simulink model "followtrajectory"  (R2022b)
settings: Solver=VariableStepAuto  StartTime=0.0  StopTime=10.0  RelTol=1e-3
libraries: robotmobilelib x1
settings Model: Creator=hp  LastModifiedBy=hp

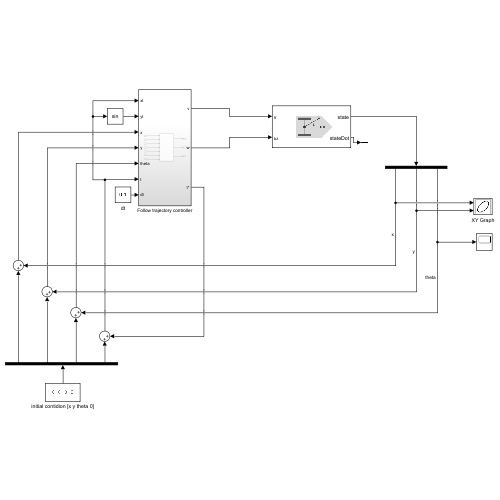
[thumbnail: Simulink's stored preview of the top-level diagram]
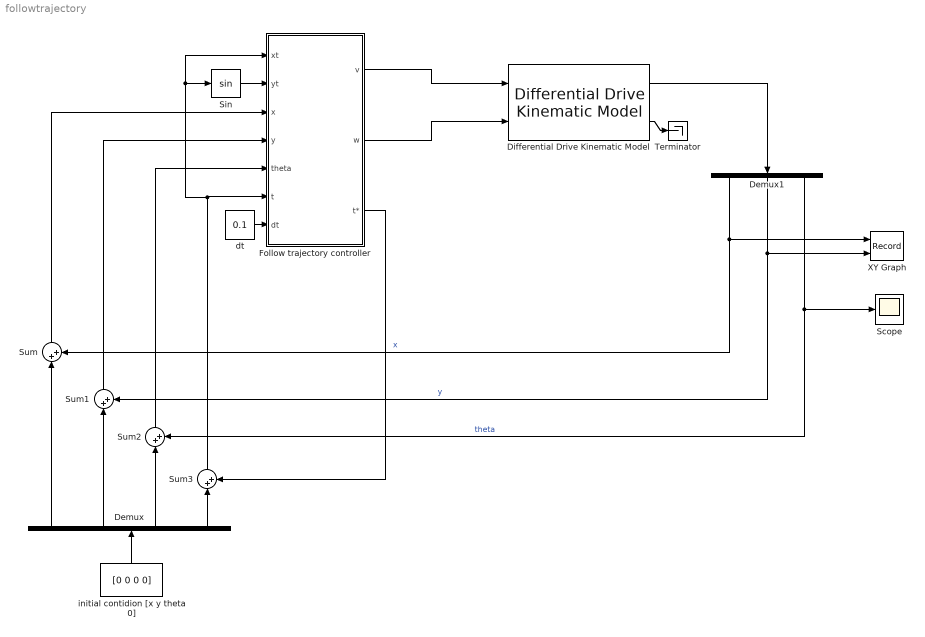
== system followtrajectory ==
  Demux : Demux
  Demux1 : Demux  Outputs=3
  Differential Drive Kinematic Model : robotmobilelib/Differential Drive Kinematic Model  VehicleInputs=Vehicle Speed & Heading Angular Velocity  WheelRadius=0.05  WheelSpeedRange=[-inf inf]  TrackWidth=0.35  InitialState=[0; 0; 0]  SimulateUsing=Interpreted execution
  Follow trajectory controller : Subsystem
  Scope : Scope
  Sin : Trigonometry
  Sum{,1..3} (4 alike) : Sum  Inputs=|++
  Terminator : Terminator
  XY Graph : Record  FileSettingsInternal="{\"entries\":[{\"content\":{\"excelSettings\":{\"content\":{},\"type\":\"Streamout.ExcelSettings\"}},\"type\":\"Streamout.FileSettingStorage\",\"uuid\":\"fe540847-13db-430f-a3f9-43ab5f5fba02\"}],\"packageUris\":[\"http://schema.mathworks.com/mf0/streamout_blocks/R2020a\"],\"version\":\"1.0\"}"  Layout=[1 1]  SignalsInternal="{\"entries\":[{\"content\":{\"signals\":[{\"content\":{\"blockPath\":[\"followtrajectory/XY Graph\"],\"channel\":[],\"dimensions\":[1],\"domain\":\"followtrajectory/XY Graph\",\"lineColor\":\"#a2142f\",\"plots\":[1],\"port\":1,\"sid\":[\"\"],\"signalID\":61,\"signalName\":\"x\"},\"type\":\"RecordBlkView.Signal\",\"uuid\":\"e5278b7b-a4bb-4301-85b3-8e4fea13731b\"},{\"content\":{\"blockPath\":[\"followtrajectory/XY Graph\"],\"channel\":[],\"dimensions\":[1],\"domain\":\"followtrajectory/XY Graph\",\"lineColor\":\"#139fff\",\"plots\":[1],\"port\":2,\"sid\":[\"\"],\"signalID\":65,\"signalName\":\"y\"},\"type\":\"RecordBlkView.Signal\",\"uuid\":\"e49be718-dbc1-456e-9503-dbe46247d26a\"}]},\"type\":\"RecordBlkView.InputSignals\",\"uuid\":\"734c241f-ef99-469e-9d0b-6cb9b84b9d56\"}],\"packageUris\":[\"http://schema.mathworks.com/mf0/streamout_blocks/R2020a\"],\"version\":\"1.0\"}"  VisualizationBindings="{\"xyplotplugin\":{\"info\":[{\"series\":[{\"bindingParametersList\":[{\"parameter\":\"X-Axis\",\"signalID\":61,\"signalName\":\"x\"},{\"parameter\":\"Y-Axis\",\"signalID\":65,\"signalName\":\"y\"}],\"seriesID\":15823}],\"subplotID\":1}]}}"  CompatibilityTag=XY
  dt : Constant  Value=0.1
  initial contidion [x y theta 0] : Constant  Value=[0 0 0 0]
  wires:
  Differential Drive Kinematic Model/2 -> Terminator/1
  Follow trajectory controller/1(v) -> Differential Drive Kinematic Model/1
  Follow trajectory controller/2(w) -> Differential Drive Kinematic Model/2
  initial contidion [x y theta 0]/1 -> Demux/1
  Differential Drive Kinematic Model/1 -> Demux1/1
  Demux/1 -> Sum/1
  Demux/2 -> Sum1/1
  Demux/3 -> Sum2/1
  Demux1/1 -> XY Graph/1, Sum/2  "x"
  Demux1/2 -> XY Graph/2, Sum1/2  "y"
  Demux1/3 -> Scope/1, Sum2/2  "theta"
  Sum/1 -> Follow trajectory controller/3(x)
  Sum1/1 -> Follow trajectory controller/4(y)
  Sum2/1 -> Follow trajectory controller/5(theta)
  dt/1 -> Follow trajectory controller/7(dt)
  Sin/1 -> Follow trajectory controller/2(yt)
  Demux/4 -> Sum3/1
  Follow trajectory controller/3(t*) -> Sum3/2
  Sum3/1 -> Follow trajectory controller/1(xt), Sin/1, Follow trajectory controller/6(t)

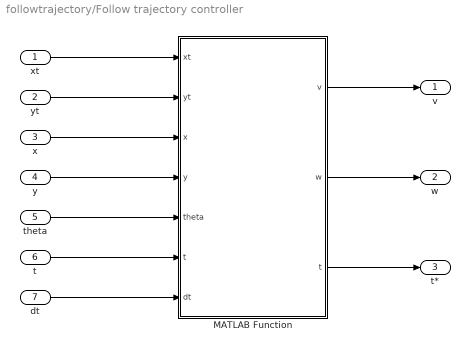
== system followtrajectory/Follow trajectory controller ==
  xt : Inport
  yt : Inport  Port=2
  x : Inport  Port=3
  y : Inport  Port=4
  theta : Inport  Port=5
  t : Inport  Port=6
  dt : Inport  Port=7
  MATLAB Function : MATLAB Function  TreatAsAtomicUnit=on
  v : Outport
  w : Outport  Port=2
  t* : Outport  Port=3
  wires:
  xt/1 -> MATLAB Function/1(xt)
  yt/1 -> MATLAB Function/2(yt)
  x/1 -> MATLAB Function/3(x)
  y/1 -> MATLAB Function/4(y)
  theta/1 -> MATLAB Function/5(theta)
  t/1 -> MATLAB Function/6("t ")
  dt/1 -> MATLAB Function/7(dt)
  MATLAB Function/1(v) -> v/1
  MATLAB Function/2(w) -> w/1
  MATLAB Function/3(t) -> t*/1

== matlab function followtrajectory/Follow trajectory controller/MATLAB Function ==
  data: xt input; v output; yt input; x input; y input; theta input; t input; dt input; w output; t output
function [v, w, t] = fcn(xt, yt, x, y, theta, t, dt)
    % Girişler:
    % xt, yt - Takip edilecek yolun x ve y koordinatları (hedef)
    % x, y - Robotun mevcut x ve y koordinatları
    % theta - Robotun mevcut yönü (açısı)
    % t - Geçen süre
    % dt - Zaman adımı
    
    d = 0.5; % Takip mesafesi (m)
    
    Kv = 1.5;
    Ki = 1.5;
    Kh = 1.5;

    e = sqrt((xt - x)^2 + (yt - y)^2) - d;
    theta_g = atan2(yt-y,xt-x);
    
    v = Kv*e + Ki*(e*t-e*(t-dt));
    w = Kh*(atan2(sin(theta_g - theta), cos(theta_g-theta)));
    t = t + dt;
end
